simulink model "gm_sampleModel17924_sub"  (R2023b)
settings: Solver=VariableStepAuto  StartTime=0.0  StopTime=10.0  RelTol=1e-3
libraries: hdlsllib x3, simulink x2
settings Model: Creator=Tsmc  LastModifiedBy=Tsmc
settings OptimizationCC: BlockReduction=off  ConditionallyExecuteInputs=off
settings DebuggingCC: InheritedTsInSrcMsg=none

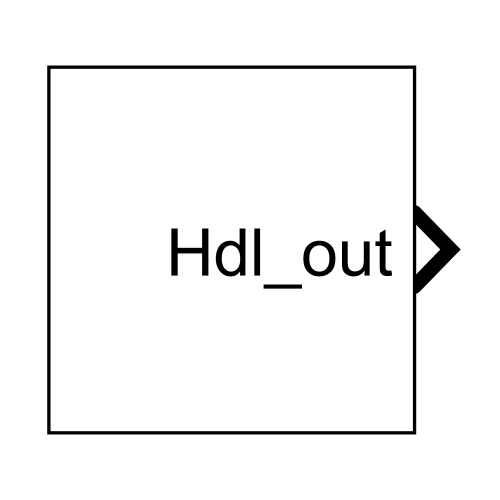
[thumbnail: Simulink's stored preview of the top-level diagram]
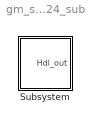
== system gm_sampleModel17924_sub ==
  Subsystem : Subsystem

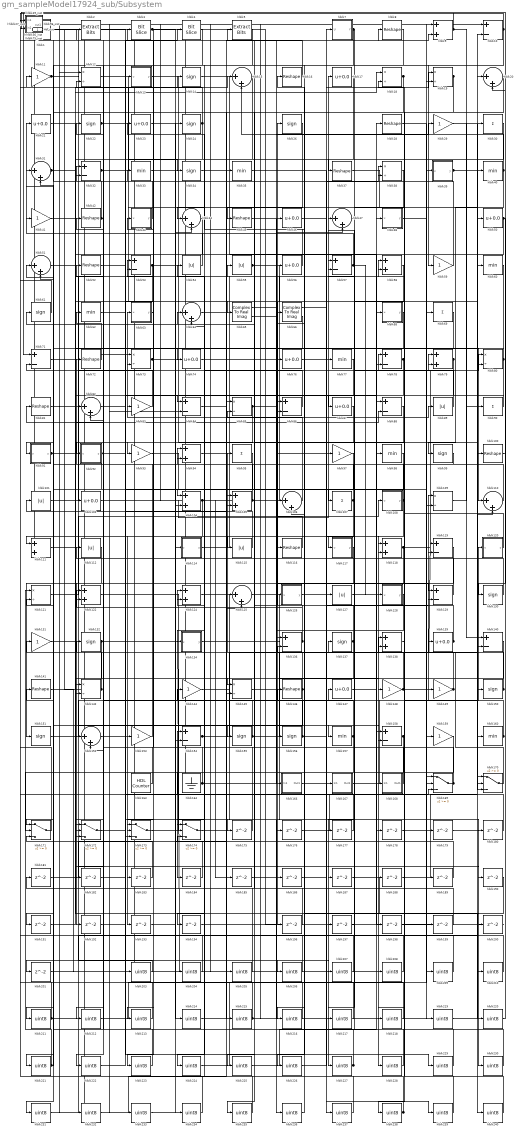
== system gm_sampleModel17924_sub/Subsystem ==
  hlblk1 : Subsystem  mask(Detect Rise Nonnegative){vinit=double(0), InputProcessing=Elements as channels (sample based), OutDataTypeStr=uint8}
      mask prompts: vinit "Simulink:masks:InitialCondition_MP"; InputProcessing "Simulink:masks:InputProcessing_MP"; OutDataTypeStr "Simulink:masks:OutputDataType_MP"
      mask help: Simulink:masks:DetectRiseNonnegative_MD
      mask init:
      | InputProcessing = 'Elements as channels (sample based)';
      | OutDataTypeStr = 'uint8';
      | vinit = double(0);
      mask TypeOptions InputProcessing: Simulink:masks:ColumnsAsChannelsFrameBased | Simulink:masks:ElementsAsChannelsSampleBased
      mask TypeOptions OutDataTypeStr: Simulink:masks:uint8 | Simulink:masks:boolean
      mask Display: fprintf('U >= 0\n&  NOT\nU/z >= 0')
  hlblk{10,32,53,57,71,78,84,86,88,119,129,136,140,154,158} (15 alike) : Sum  Inputs=+-  OutDataTypeStr=uint8
  hlblk{8,16,28,37,42,45,52,72,81,100,116,141,146} (13 alike) : Reshape
  hlblk{54..55,89,101,112,115,127} (7 alike) : Abs  OutDataTypeStr=uint8  SaturateOnIntegerOverflow=off
  hlblk{17,21,23,46,50,56,74,76,87,102,139,147} (12 alike) : Bias  Bias=0.0  SaturateOnIntegerOverflow=off
  hlblk{9,58,79,94,104..105,111,118,122,124,138} (11 alike) : Sum  OutDataTypeStr=uint8
  hlblk{15,20,31,44,47,51,64,82,106,110,125,152} (12 alike) : Sum  Inputs=|++  OutDataTypeStr=uint8
  hlblk{30,69,90,95,107} (5 alike) : Sum  Inputs=+  OutDataTypeStr=uint8
  hlblk108 : Subsystem  mask(Real World Value Increment){}
      mask help: Simulink:masks:RealWorldValueIncrement_MD
      mask Display: disp('V++')
  hlblk{12,18..19,38,73,80,85,109,121,142,145} (11 alike) : Product  Inputs=*/  OutDataTypeStr=uint8  RndMeth=Zero  SaturateOnIntegerOverflow=on
  hlblk{11,29,41,59,83,93,97,131,144,148..149,153,159} (13 alike) : Gain  OutDataTypeStr=uint8
  hlblk113_inst : Subsystem
  hlblk114 : Subsystem  mask(Real World Value Increment){}
      mask help: Simulink:masks:RealWorldValueIncrement_MD
      mask Display: disp('V++')
  hlblk117 : Subsystem  mask(Real World Value Increment){}
      mask help: Simulink:masks:RealWorldValueIncrement_MD
      mask Display: disp('V++')
  hlblk120 : Subsystem  mask(Real World Value Increment){}
      mask help: Simulink:masks:RealWorldValueIncrement_MD
      mask Display: disp('V++')
  hlblk126 : Subsystem  mask(Real World Value Increment){}
      mask help: Simulink:masks:RealWorldValueIncrement_MD
      mask Display: disp('V++')
  hlblk128 : Subsystem  mask(Real World Value Increment){}
      mask help: Simulink:masks:RealWorldValueIncrement_MD
      mask Display: disp('V++')
  hlblk13 : Subsystem  mask(Real World Value Increment){}
      mask help: Simulink:masks:RealWorldValueIncrement_MD
      mask Display: disp('V++')
  hlblk{14,22,24,26,34,61,99,130,132,137,150..151,155..156} (14 alike) : Signum
  hlblk133_inst : Subsystem
  hlblk134 : Subsystem  mask(Real World Value Increment){}
      mask help: Simulink:masks:RealWorldValueIncrement_MD
      mask Display: disp('V++')
  hlblk135_inst : Subsystem
  hlblk143_inst : Subsystem
  hlblk{33,35,40,60,62,77,98,157,160} (9 alike) : MinMax  OutDataTypeStr=uint8
  hlblk163 : hdlsllib/Sources/HDL Counter  CountType=Count limited  CountInit=0  CountStep=1  CountMax=25  CountFromType=Initial value  CountFrom=0  CountResetPort=off  CountLoadPort=off  CountEnbPort=off  CountDirPort=off  CountHitOutputPort=off  CountDataType=Unsigned  CountWordLen=8  CountFracLen=0  CountSampTime=1
  hlblk164 : Ground
  hlblk166 : Subsystem
  hlblk167 : Subsystem
  hlblk168 : Subsystem
  hlblk{169..174} (6 alike) : Switch  OutDataTypeStr=uint8  SaturateOnIntegerOverflow=off  InputSameDT=off
  hlblk{175..194,196..201} (26 alike) : Delay  SampleTime=1
  hlblk2 : simulink/Logic and Bit Operations/Extract Bits  bitsToExtract=Upper half  numBits=8  bitIdxRange=[0 7]  outScalingMode=Preserve fixed-point scaling
      settings: LibrarySourceBlock=|
      | hdlsllib/Logic and Bit
      | Operations/Extract Bits
  hlblk{203..240} (38 alike) : DataTypeConversion  OutDataTypeStr=uint8  SaturateOnIntegerOverflow=off  RndMeth=Floor
  hlblk25_inst : Subsystem
  hlblk27_inst : Subsystem
  hlblk3 : hdlsllib/Logic and Bit Operations/Bit Slice  lidx=7  ridx=0
  hlblk36_inst : Subsystem
  hlblk39 : Subsystem  mask(Real World Value Increment){}
      mask help: Simulink:masks:RealWorldValueIncrement_MD
      mask Display: disp('V++')
  hlblk4 : hdlsllib/Logic and Bit Operations/Bit Slice  lidx=7  ridx=0
  hlblk43 : Subsystem  mask(Real World Value Increment){}
      mask help: Simulink:masks:RealWorldValueIncrement_MD
      mask Display: disp('V++')
  hlblk48 : Subsystem  mask(Real World Value Increment){}
      mask help: Simulink:masks:RealWorldValueIncrement_MD
      mask Display: disp('V++')
  hlblk49_inst : Subsystem
  hlblk5 : simulink/Logic and Bit Operations/Extract Bits  bitsToExtract=Upper half  numBits=8  bitIdxRange=[0 7]  outScalingMode=Preserve fixed-point scaling
      settings: LibrarySourceBlock=|
      | hdlsllib/Logic and Bit
      | Operations/Extract Bits
  hlblk63 : Subsystem  mask(Real World Value Increment){}
      mask help: Simulink:masks:RealWorldValueIncrement_MD
      mask Display: disp('V++')
  hlblk65 : ComplexToRealImag
  hlblk66 : ComplexToRealImag
  hlblk68 : Subsystem  mask(Real World Value Increment){}
      mask help: Simulink:masks:RealWorldValueIncrement_MD
      mask Display: disp('V++')
  hlblk7 : Subsystem  mask(Detect Fall Negative){vinit=double(0), InputProcessing=Elements as channels (sample based), OutDataTypeStr=uint8}
      mask prompts: vinit "Simulink:masks:InitialCondition_MP"; InputProcessing "Simulink:masks:InputProcessing_MP"; OutDataTypeStr "Simulink:masks:OutputDataType_MP"
      mask help: Simulink:masks:DetectFallNegative_MD
      mask init:
      | InputProcessing = 'Elements as channels (sample based)';
      | OutDataTypeStr = 'uint8';
      | vinit = double(0);
      mask TypeOptions InputProcessing: Simulink:masks:ColumnsAsChannelsFrameBased | Simulink:masks:ElementsAsChannelsSampleBased
      mask TypeOptions OutDataTypeStr: Simulink:masks:uint8 | Simulink:masks:boolean
      mask Display: fprintf('U < 0\n&  NOT\nU/z < 0')
  hlblk75_inst : Subsystem
  hlblk91 : Subsystem  mask(Real World Value Increment){}
      mask help: Simulink:masks:RealWorldValueIncrement_MD
      mask Display: disp('V++')
  hlblk92 : Subsystem  mask(Real World Value Increment){}
      mask help: Simulink:masks:RealWorldValueIncrement_MD
      mask Display: disp('V++')
  hlblk96_inst : Subsystem
  Hdl_out : Outport  OutDataTypeStr=uint8  SampleTime=1
  wires:
  hlblk1/1(Y) -> hlblk206/1
  hlblk10/1 -> hlblk71/1, hlblk106/2, hlblk59/1
  hlblk100/1 -> hlblk75_inst/2(in2)
  hlblk101/1 -> hlblk55/1
  hlblk102/1 -> hlblk17/1
  hlblk104/1 -> hlblk111/1, hlblk185/1
  hlblk105/1 -> hlblk94/1, hlblk58/1
  hlblk106/1 -> hlblk63/1(u)
  hlblk107/1 -> hlblk31/2, hlblk193/1
  hlblk108/1(y) -> hlblk72/1, hlblk228/1
  hlblk109/1 -> hlblk30/1
  hlblk11/1 -> hlblk214/1, hlblk110/1
  hlblk110/1 -> hlblk5/1
  hlblk111/1 -> hlblk157/1
  hlblk112/1 -> hlblk151/1
  hlblk113_inst/1(out1) -> hlblk205/1
  hlblk114/1(y) -> hlblk48/1(u)
  hlblk115/1 -> hlblk51/1
  hlblk116/1 -> hlblk26/1
  hlblk117/1(y) -> hlblk183/1
  hlblk118/1 -> hlblk196/1, hlblk80/1
  hlblk119/1 -> hlblk192/1
  hlblk12/1 -> hlblk176/1
  hlblk120/1(y) -> hlblk18/2
  hlblk121/1 -> hlblk108/1(u)
  hlblk122/1 -> hlblk175/1
  hlblk124/1 -> hlblk227/1
  hlblk125/1 -> hlblk230/1
  hlblk126/1(y) -> hlblk7/1(U)
  hlblk127/1 -> hlblk68/1(u)
  hlblk128/1(y) -> hlblk136/1
  hlblk129/1 -> hlblk53/1
  hlblk13/1(y) -> hlblk170/2
  hlblk130/1 -> hlblk109/1
  hlblk131/1 -> hlblk187/1
  hlblk132/1 -> hlblk204/1, hlblk172/3
  hlblk133_inst/1(out1) -> hlblk111/2, hlblk167/1(In1)
  hlblk134/1(y) -> hlblk148/1
  hlblk135_inst/1(out1) -> hlblk12/1
  hlblk136/1 -> hlblk86/2, hlblk122/1
  hlblk137/1 -> hlblk235/1, hlblk83/1
  hlblk138/1 -> hlblk238/1
  hlblk139/1 -> hlblk61/1, hlblk112/1
  hlblk14/1 -> hlblk198/1
  hlblk140/1 -> hlblk142/2
  hlblk141/1 -> hlblk203/1
  hlblk142/1 -> hlblk131/1, Hdl_out/1
  hlblk143_inst/1(out1) -> hlblk84/2, hlblk234/1, hlblk220/1
  hlblk144/1 -> hlblk236/1
  hlblk145/1 -> hlblk28/1
  hlblk146/1 -> hlblk46/1, hlblk171/1, hlblk43/1(u)
  hlblk147/1 -> hlblk88/1
  hlblk148/1 -> hlblk119/1, hlblk95/1
  hlblk149/1 -> hlblk22/1, hlblk119/2
  hlblk15/1 -> hlblk194/1
  hlblk150/1 -> hlblk142/1, hlblk73/2
  hlblk151/1 -> hlblk120/1(u)
  hlblk152/1 -> hlblk153/1
  hlblk153/1 -> hlblk2/1
  hlblk154/1 -> hlblk147/1, hlblk140/2
  hlblk155/1 -> hlblk32/1, hlblk152/1, hlblk40/1
  hlblk156/1 -> hlblk3/1, hlblk129/2, hlblk38/1
  hlblk157/1 -> hlblk184/1, hlblk126/1(u)
  hlblk158/1 -> hlblk173/2, hlblk171/2
  hlblk159/1 -> hlblk223/1
  hlblk16/1 -> hlblk135_inst/2(in2)
  hlblk160/1 -> hlblk58/2, hlblk149/1
  hlblk163/1 -> hlblk52/1
  hlblk164/1 -> hlblk53/2, hlblk237/1
  hlblk166/1(Out1) -> hlblk19/1
  hlblk167/1(Out1) -> hlblk19/2
  hlblk168/1(Out1) -> hlblk47/1
  hlblk169/1 -> hlblk82/2, hlblk81/1, hlblk16/1
  hlblk17/1 -> hlblk37/1
  hlblk170/1 -> hlblk139/1
  hlblk171/1 -> hlblk143_inst/1(in1)
  hlblk172/1 -> hlblk105/1
  hlblk173/1 -> hlblk150/1
  hlblk174/1 -> hlblk89/1
  hlblk175/1 -> hlblk27_inst/2(in2)
  hlblk176/1 -> hlblk9/1
  hlblk177/1 -> hlblk154/1
  hlblk178/1 -> hlblk170/1
  hlblk179/1 -> hlblk210/1
  hlblk18/1 -> hlblk51/2, hlblk145/1
  hlblk180/1 -> hlblk25_inst/2(in2)
  hlblk181/1 -> hlblk105/2
  hlblk182/1 -> hlblk169/3
  hlblk183/1 -> hlblk121/2
  hlblk184/1 -> hlblk174/3
  hlblk185/1 -> hlblk86/1
  hlblk186/1 -> hlblk79/1
  hlblk187/1 -> hlblk240/1
  hlblk188/1 -> hlblk110/2
  hlblk189/1 -> hlblk174/2
  hlblk19/1 -> hlblk104/1, hlblk145/2
  hlblk190/1 -> hlblk216/1
  hlblk191/1 -> hlblk88/2
  hlblk192/1 -> hlblk80/2
  hlblk193/1 -> hlblk78/1
  hlblk194/1 -> hlblk47/2
  hlblk196/1 -> hlblk71/2
  hlblk197/1 -> hlblk57/1
  hlblk198/1 -> hlblk169/2
  hlblk199/1 -> hlblk85/2
  hlblk2/1 -> hlblk186/1
  hlblk20/1 -> hlblk218/1
  hlblk200/1 -> hlblk1/1(U)
  hlblk201/1 -> hlblk207/1
  hlblk203/1 -> hlblk201/1
  hlblk204/1 -> hlblk141/1
  hlblk205/1 -> hlblk85/1
  hlblk206/1 -> hlblk113_inst/1(in1)
  hlblk207/1 -> hlblk113_inst/2(in2)
  hlblk208/1 -> hlblk96_inst/1(in1)
  hlblk209/1 -> hlblk49_inst/1(in1)
  hlblk21/1 -> hlblk102/1
  hlblk210/1 -> hlblk49_inst/2(in2)
  hlblk211/1 -> hlblk24/1, hlblk133_inst/2(in2), hlblk10/2
  hlblk212/1 -> hlblk69/1
  hlblk213/1 -> hlblk143_inst/2(in2)
  hlblk214/1 -> hlblk98/1
  hlblk215/1 -> hlblk171/3, hlblk169/1
  hlblk216/1 -> hlblk64/1
  hlblk217/1 -> hlblk64/2
  hlblk218/1 -> hlblk135_inst/1(in1)
  hlblk219/1 -> hlblk20/1
  hlblk22/1 -> hlblk34/1, hlblk199/1
  hlblk220/1 -> hlblk20/2
  hlblk221/1 -> hlblk101/1, hlblk121/1
  hlblk222/1 -> hlblk4/1
  hlblk223/1 -> hlblk132/1
  hlblk224/1 -> hlblk159/1
  hlblk225/1 -> hlblk168/1(In1)
  hlblk226/1 -> hlblk77/1
  hlblk227/1 -> hlblk42/1, hlblk181/1
  hlblk228/1 -> hlblk124/1
  hlblk229/1 -> hlblk124/2
  hlblk23/1 -> hlblk44/2
  hlblk230/1 -> hlblk137/1
  hlblk231/1 -> hlblk125/1
  hlblk232/1 -> hlblk125/2
  hlblk233/1 -> hlblk114/1(u)
  hlblk234/1 -> hlblk36_inst/1(in1)
  hlblk235/1 -> hlblk36_inst/2(in2)
  hlblk236/1 -> hlblk146/1
  hlblk237/1 -> hlblk144/1
  hlblk238/1 -> hlblk66/1, hlblk136/2
  hlblk239/1 -> hlblk138/1
  hlblk24/1 -> hlblk96_inst/2(in2), hlblk32/2
  hlblk240/1 -> hlblk138/2
  hlblk25_inst/1(out1) -> hlblk232/1, hlblk10/1
  hlblk26/1 -> hlblk45/1
  hlblk27_inst/1(out1) -> hlblk13/1(u), hlblk35/1
  hlblk28/1 -> hlblk219/1
  hlblk29/1 -> hlblk60/1
  hlblk3/1 -> hlblk173/1, hlblk158/2
  hlblk30/1 -> hlblk172/1
  hlblk31/1 -> hlblk15/1, hlblk91/1(u)
  hlblk32/1 -> hlblk209/1, hlblk14/1
  hlblk33/1 -> hlblk190/1
  hlblk34/1 -> hlblk78/2
  hlblk35/1 -> hlblk239/1
  hlblk36_inst/1(out1) -> hlblk233/1
  hlblk37/1 -> hlblk160/1
  hlblk38/1 -> hlblk177/1
  hlblk39/1(y) -> hlblk50/1, hlblk90/1
  hlblk4/1 -> hlblk221/1
  hlblk40/1 -> hlblk99/1, hlblk15/2
  hlblk41/1 -> hlblk200/1
  hlblk42/1 -> hlblk152/2, hlblk133_inst/1(in1), hlblk12/2
  hlblk43/1(y) -> hlblk75_inst/1(in1)
  hlblk44/1 -> hlblk222/1
  hlblk45/1 -> hlblk156/1
  hlblk46/1 -> hlblk38/2
  hlblk47/1 -> hlblk217/1
  hlblk48/1(y) -> hlblk179/1
  hlblk49_inst/1(out1) -> hlblk208/1
  hlblk5/1 -> hlblk44/1
  hlblk50/1 -> hlblk172/2, hlblk130/1, hlblk118/2
  hlblk51/1 -> hlblk84/1
  hlblk52/1 -> hlblk65/1
  hlblk53/1 -> hlblk170/3, hlblk122/2
  hlblk54/1 -> hlblk21/1
  hlblk55/1 -> hlblk158/1, hlblk100/1, hlblk189/1
  hlblk56/1 -> hlblk23/1
  hlblk57/1 -> hlblk41/1, hlblk128/1(u)
  hlblk58/1 -> hlblk197/1
  hlblk59/1 -> hlblk11/1
  hlblk60/1 -> hlblk104/2
  hlblk61/1 -> hlblk25_inst/1(in1)
  hlblk62/1 -> hlblk180/1
  hlblk63/1(y) -> hlblk33/1
  hlblk64/1 -> hlblk215/1
  hlblk65/1 -> hlblk97/1
  hlblk65/2 -> hlblk29/1
  hlblk66/1 -> hlblk127/1
  hlblk66/2 -> hlblk224/1
  hlblk68/1(y) -> hlblk174/1
  hlblk69/1 -> hlblk211/1
  hlblk7/1(Y) -> hlblk182/1, hlblk117/1(u)
  hlblk71/1 -> hlblk76/1
  hlblk72/1 -> hlblk62/1
  hlblk73/1 -> hlblk188/1, hlblk166/1(In1)
  hlblk74/1 -> hlblk107/1
  hlblk75_inst/1(out1) -> hlblk106/1, hlblk73/1
  hlblk76/1 -> hlblk118/1
  hlblk77/1 -> hlblk225/1
  hlblk78/1 -> hlblk173/3, hlblk154/2
  hlblk79/1 -> hlblk116/1, hlblk115/1
  hlblk8/1 -> hlblk93/1
  hlblk80/1 -> hlblk74/1, hlblk134/1(u)
  hlblk81/1 -> hlblk39/1(u)
  hlblk82/1 -> hlblk109/2
  hlblk83/1 -> hlblk31/1
  hlblk84/1 -> hlblk8/1
  hlblk85/1 -> hlblk9/2, hlblk129/1, hlblk92/1(u)
  hlblk86/1 -> hlblk54/1
  hlblk87/1 -> hlblk155/1
  hlblk88/1 -> hlblk226/1
  hlblk89/1 -> hlblk57/2
  hlblk9/1 -> hlblk27_inst/1(in1), hlblk140/1
  hlblk90/1 -> hlblk87/1
  hlblk91/1(y) -> hlblk56/1, hlblk18/1
  hlblk92/1(y) -> hlblk231/1, hlblk229/1
  hlblk93/1 -> hlblk178/1
  hlblk94/1 -> hlblk79/2
  hlblk95/1 -> hlblk191/1
  hlblk96_inst/1(out1) -> hlblk82/1
  hlblk97/1 -> hlblk212/1
  hlblk98/1 -> hlblk213/1
  hlblk99/1 -> hlblk94/2

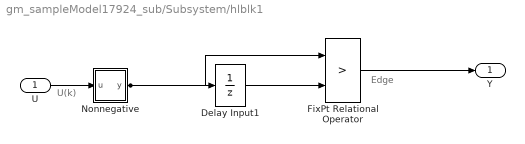
== system gm_sampleModel17924_sub/Subsystem/hlblk1 ==
  note: U(k)
  note: Edge
  U : Inport  OutDataTypeStr=uint8  SampleTime=1
  Delay Input1 : UnitDelay  Description=Store in Global RAM  DisableCoverage=on  InitialCondition=vinit  SampleTime=-1  HasFrameUpgradeWarning=on
  FixPt Relational Operator : RelationalOperator  Operator=>  OutDataTypeStr=fixdt(0, 8)  ZeroCross=off  InputSameDT=off
  Nonnegative : Subsystem  mask(Compare To Zero){relop=>=, OutDataTypeStr=boolean, ZeroCross=off}
      mask prompts: relop "Simulink:masks:Operator_MP"; OutDataTypeStr "Simulink:masks:OutputDataType_MP"; ZeroCross "Simulink:masks:EnableZerocrossingDetection_MP"
      mask help: Simulink:masks:CompareToZero_MD
      mask init:
      | OutDataTypeStr = 'boolean';
      | ZeroCross = 'off';
      | blkName = 'sampleModel17924_sub/Subsystem/hlblk1/Nonnegative';
      | relop = '>=';
      | setValue = 'boolean';
      mask TypeOptions relop: == | ~= | < | <= | >= | >
      mask TypeOptions OutDataTypeStr: Simulink:masks:uint8 | Simulink:masks:boolean
      mask Callback ZeroCross: sl('zeroCrossEnable', gcbh);
      mask Display: disp([relop,' 0'])
  Y : Outport  SampleTime=1
  wires:
  U/1 -> Nonnegative/1(u)
  Delay Input1/1 -> FixPt Relational Operator/2
  FixPt Relational Operator/1 -> Y/1
  Nonnegative/1(y) -> FixPt Relational Operator/1, Delay Input1/1

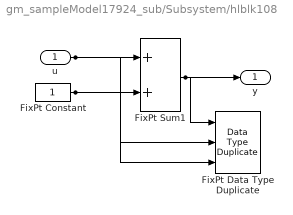
== system gm_sampleModel17924_sub/Subsystem/hlblk108 ==
  u : Inport  OutDataTypeStr=uint8  SampleTime=1
  FixPt Constant : Constant  DisableCoverage=on  OutDataTypeStr=Inherit: Inherit via back propagation  SampleTime=-1
  FixPt Data Type Duplicate : DataTypeDuplicate  DisableCoverage=on  NumInputPorts=3
  FixPt Sum1 : Sum  OutDataTypeStr=Inherit: Inherit via back propagation  InputSameDT=on  LockScale=on
  y : Outport  SampleTime=1
  wires:
  u/1 -> FixPt Sum1/1, FixPt Data Type Duplicate/2
  FixPt Constant/1 -> FixPt Sum1/2, FixPt Data Type Duplicate/3
  FixPt Sum1/1 -> FixPt Data Type Duplicate/1, y/1

== system gm_sampleModel17924_sub/Subsystem/hlblk113_inst ==
  in1 : Inport  OutDataTypeStr=uint8  SampleTime=1
  in2 : Inport  Port=2  OutDataTypeStr=uint8  SampleTime=1
  mul_hlblk113_dotp_mulcomp : Product  Inputs=**  OutDataTypeStr=uint8  SampleTime=1
  out1 : Outport  OutDataTypeStr=uint8  SampleTime=1
  wires:
  in1/1 -> mul_hlblk113_dotp_mulcomp/1
  in2/1 -> mul_hlblk113_dotp_mulcomp/2
  mul_hlblk113_dotp_mulcomp/1 -> out1/1

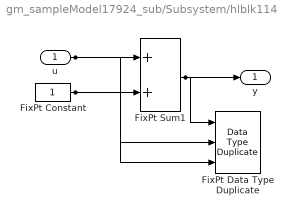
== system gm_sampleModel17924_sub/Subsystem/hlblk114 ==
  u : Inport  OutDataTypeStr=uint8  SampleTime=1
  FixPt Constant : Constant  DisableCoverage=on  OutDataTypeStr=Inherit: Inherit via back propagation  SampleTime=-1
  FixPt Data Type Duplicate : DataTypeDuplicate  DisableCoverage=on  NumInputPorts=3
  FixPt Sum1 : Sum  OutDataTypeStr=Inherit: Inherit via back propagation  InputSameDT=on  LockScale=on
  y : Outport  SampleTime=1
  wires:
  u/1 -> FixPt Sum1/1, FixPt Data Type Duplicate/2
  FixPt Constant/1 -> FixPt Sum1/2, FixPt Data Type Duplicate/3
  FixPt Sum1/1 -> FixPt Data Type Duplicate/1, y/1

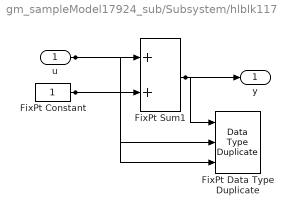
== system gm_sampleModel17924_sub/Subsystem/hlblk117 ==
  u : Inport  OutDataTypeStr=uint8  SampleTime=1
  FixPt Constant : Constant  DisableCoverage=on  OutDataTypeStr=Inherit: Inherit via back propagation  SampleTime=-1
  FixPt Data Type Duplicate : DataTypeDuplicate  DisableCoverage=on  NumInputPorts=3
  FixPt Sum1 : Sum  OutDataTypeStr=Inherit: Inherit via back propagation  InputSameDT=on  LockScale=on
  y : Outport  SampleTime=1
  wires:
  u/1 -> FixPt Sum1/1, FixPt Data Type Duplicate/2
  FixPt Constant/1 -> FixPt Sum1/2, FixPt Data Type Duplicate/3
  FixPt Sum1/1 -> FixPt Data Type Duplicate/1, y/1

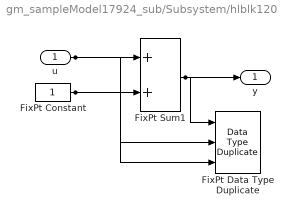
== system gm_sampleModel17924_sub/Subsystem/hlblk120 ==
  u : Inport  OutDataTypeStr=uint8  SampleTime=1
  FixPt Constant : Constant  DisableCoverage=on  OutDataTypeStr=Inherit: Inherit via back propagation  SampleTime=-1
  FixPt Data Type Duplicate : DataTypeDuplicate  DisableCoverage=on  NumInputPorts=3
  FixPt Sum1 : Sum  OutDataTypeStr=Inherit: Inherit via back propagation  InputSameDT=on  LockScale=on
  y : Outport  SampleTime=1
  wires:
  u/1 -> FixPt Sum1/1, FixPt Data Type Duplicate/2
  FixPt Constant/1 -> FixPt Sum1/2, FixPt Data Type Duplicate/3
  FixPt Sum1/1 -> FixPt Data Type Duplicate/1, y/1

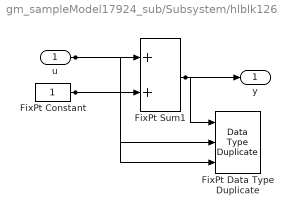
== system gm_sampleModel17924_sub/Subsystem/hlblk126 ==
  u : Inport  OutDataTypeStr=uint8  SampleTime=1
  FixPt Constant : Constant  DisableCoverage=on  OutDataTypeStr=Inherit: Inherit via back propagation  SampleTime=-1
  FixPt Data Type Duplicate : DataTypeDuplicate  DisableCoverage=on  NumInputPorts=3
  FixPt Sum1 : Sum  OutDataTypeStr=Inherit: Inherit via back propagation  InputSameDT=on  LockScale=on
  y : Outport  SampleTime=1
  wires:
  u/1 -> FixPt Sum1/1, FixPt Data Type Duplicate/2
  FixPt Constant/1 -> FixPt Sum1/2, FixPt Data Type Duplicate/3
  FixPt Sum1/1 -> FixPt Data Type Duplicate/1, y/1

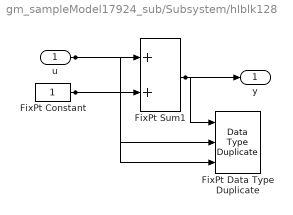
== system gm_sampleModel17924_sub/Subsystem/hlblk128 ==
  u : Inport  OutDataTypeStr=uint8  SampleTime=1
  FixPt Constant : Constant  DisableCoverage=on  OutDataTypeStr=Inherit: Inherit via back propagation  SampleTime=-1
  FixPt Data Type Duplicate : DataTypeDuplicate  DisableCoverage=on  NumInputPorts=3
  FixPt Sum1 : Sum  OutDataTypeStr=Inherit: Inherit via back propagation  InputSameDT=on  LockScale=on
  y : Outport  SampleTime=1
  wires:
  u/1 -> FixPt Sum1/1, FixPt Data Type Duplicate/2
  FixPt Constant/1 -> FixPt Sum1/2, FixPt Data Type Duplicate/3
  FixPt Sum1/1 -> FixPt Data Type Duplicate/1, y/1

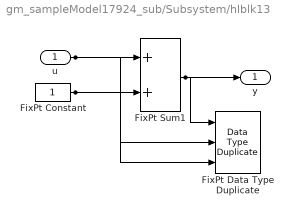
== system gm_sampleModel17924_sub/Subsystem/hlblk13 ==
  u : Inport  OutDataTypeStr=uint8  SampleTime=1
  FixPt Constant : Constant  DisableCoverage=on  OutDataTypeStr=Inherit: Inherit via back propagation  SampleTime=-1
  FixPt Data Type Duplicate : DataTypeDuplicate  DisableCoverage=on  NumInputPorts=3
  FixPt Sum1 : Sum  OutDataTypeStr=Inherit: Inherit via back propagation  InputSameDT=on  LockScale=on
  y : Outport  SampleTime=1
  wires:
  u/1 -> FixPt Sum1/1, FixPt Data Type Duplicate/2
  FixPt Constant/1 -> FixPt Sum1/2, FixPt Data Type Duplicate/3
  FixPt Sum1/1 -> FixPt Data Type Duplicate/1, y/1

== system gm_sampleModel17924_sub/Subsystem/hlblk133_inst ==
  in1 : Inport  OutDataTypeStr=uint8  SampleTime=1
  in2 : Inport  Port=2  OutDataTypeStr=uint8  SampleTime=1
  mul_hlblk133_dotp_mulcomp : Product  Inputs=**  OutDataTypeStr=uint8  SampleTime=1
  out1 : Outport  OutDataTypeStr=uint8  SampleTime=1
  wires:
  in1/1 -> mul_hlblk133_dotp_mulcomp/1
  in2/1 -> mul_hlblk133_dotp_mulcomp/2
  mul_hlblk133_dotp_mulcomp/1 -> out1/1

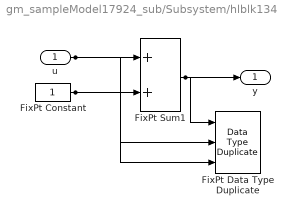
== system gm_sampleModel17924_sub/Subsystem/hlblk134 ==
  u : Inport  OutDataTypeStr=uint8  SampleTime=1
  FixPt Constant : Constant  DisableCoverage=on  OutDataTypeStr=Inherit: Inherit via back propagation  SampleTime=-1
  FixPt Data Type Duplicate : DataTypeDuplicate  DisableCoverage=on  NumInputPorts=3
  FixPt Sum1 : Sum  OutDataTypeStr=Inherit: Inherit via back propagation  InputSameDT=on  LockScale=on
  y : Outport  SampleTime=1
  wires:
  u/1 -> FixPt Sum1/1, FixPt Data Type Duplicate/2
  FixPt Constant/1 -> FixPt Sum1/2, FixPt Data Type Duplicate/3
  FixPt Sum1/1 -> FixPt Data Type Duplicate/1, y/1

== system gm_sampleModel17924_sub/Subsystem/hlblk135_inst ==
  in1 : Inport  OutDataTypeStr=uint8  SampleTime=1
  in2 : Inport  Port=2  OutDataTypeStr=uint8  SampleTime=1
  mul_hlblk135_dotp_mulcomp : Product  Inputs=**  OutDataTypeStr=uint8  SampleTime=1
  out1 : Outport  OutDataTypeStr=uint8  SampleTime=1
  wires:
  in1/1 -> mul_hlblk135_dotp_mulcomp/1
  in2/1 -> mul_hlblk135_dotp_mulcomp/2
  mul_hlblk135_dotp_mulcomp/1 -> out1/1

== system gm_sampleModel17924_sub/Subsystem/hlblk143_inst ==
  in1 : Inport  OutDataTypeStr=uint8  SampleTime=1
  in2 : Inport  Port=2  OutDataTypeStr=uint8  SampleTime=1
  mul_hlblk143_dotp_mulcomp : Product  Inputs=**  OutDataTypeStr=uint8  SampleTime=1
  out1 : Outport  OutDataTypeStr=uint8  SampleTime=1
  wires:
  in1/1 -> mul_hlblk143_dotp_mulcomp/1
  in2/1 -> mul_hlblk143_dotp_mulcomp/2
  mul_hlblk143_dotp_mulcomp/1 -> out1/1

== system gm_sampleModel17924_sub/Subsystem/hlblk166 ==
  In1 : Inport  OutDataTypeStr=uint8  PortDimensions=1  SampleTime=1
  Out1 : Outport  SampleTime=1
  wires:
  In1/1 -> Out1/1

== system gm_sampleModel17924_sub/Subsystem/hlblk167 ==
  In1 : Inport  OutDataTypeStr=uint8  PortDimensions=1  SampleTime=1
  Out1 : Outport  SampleTime=1
  wires:
  In1/1 -> Out1/1

== system gm_sampleModel17924_sub/Subsystem/hlblk168 ==
  In1 : Inport  OutDataTypeStr=uint8  PortDimensions=1  SampleTime=1
  Out1 : Outport  SampleTime=1
  wires:
  In1/1 -> Out1/1

== system gm_sampleModel17924_sub/Subsystem/hlblk25_inst ==
  in1 : Inport  OutDataTypeStr=uint8  SampleTime=1
  in2 : Inport  Port=2  OutDataTypeStr=uint8  SampleTime=1
  mul_hlblk25_dotp_mulcomp : Product  Inputs=**  OutDataTypeStr=uint8  SampleTime=1
  out1 : Outport  OutDataTypeStr=uint8  SampleTime=1
  wires:
  in1/1 -> mul_hlblk25_dotp_mulcomp/1
  in2/1 -> mul_hlblk25_dotp_mulcomp/2
  mul_hlblk25_dotp_mulcomp/1 -> out1/1

== system gm_sampleModel17924_sub/Subsystem/hlblk27_inst ==
  in1 : Inport  OutDataTypeStr=uint8  SampleTime=1
  in2 : Inport  Port=2  OutDataTypeStr=uint8  SampleTime=1
  mul_hlblk27_dotp_mulcomp : Product  Inputs=**  OutDataTypeStr=uint8  SampleTime=1
  out1 : Outport  OutDataTypeStr=uint8  SampleTime=1
  wires:
  in1/1 -> mul_hlblk27_dotp_mulcomp/1
  in2/1 -> mul_hlblk27_dotp_mulcomp/2
  mul_hlblk27_dotp_mulcomp/1 -> out1/1

== system gm_sampleModel17924_sub/Subsystem/hlblk36_inst ==
  in1 : Inport  OutDataTypeStr=uint8  SampleTime=1
  in2 : Inport  Port=2  OutDataTypeStr=uint8  SampleTime=1
  mul_hlblk36_dotp_mulcomp : Product  Inputs=**  OutDataTypeStr=uint8  SampleTime=1
  out1 : Outport  OutDataTypeStr=uint8  SampleTime=1
  wires:
  in1/1 -> mul_hlblk36_dotp_mulcomp/1
  in2/1 -> mul_hlblk36_dotp_mulcomp/2
  mul_hlblk36_dotp_mulcomp/1 -> out1/1

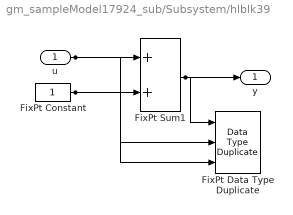
== system gm_sampleModel17924_sub/Subsystem/hlblk39 ==
  u : Inport  OutDataTypeStr=uint8  SampleTime=1
  FixPt Constant : Constant  DisableCoverage=on  OutDataTypeStr=Inherit: Inherit via back propagation  SampleTime=-1
  FixPt Data Type Duplicate : DataTypeDuplicate  DisableCoverage=on  NumInputPorts=3
  FixPt Sum1 : Sum  OutDataTypeStr=Inherit: Inherit via back propagation  InputSameDT=on  LockScale=on
  y : Outport  SampleTime=1
  wires:
  u/1 -> FixPt Sum1/1, FixPt Data Type Duplicate/2
  FixPt Constant/1 -> FixPt Sum1/2, FixPt Data Type Duplicate/3
  FixPt Sum1/1 -> FixPt Data Type Duplicate/1, y/1

== system gm_sampleModel17924_sub/Subsystem/hlblk43 ==
  u : Inport  OutDataTypeStr=uint8  SampleTime=1
  FixPt Constant : Constant  DisableCoverage=on  OutDataTypeStr=Inherit: Inherit via back propagation  SampleTime=-1
  FixPt Data Type Duplicate : DataTypeDuplicate  DisableCoverage=on  NumInputPorts=3
  FixPt Sum1 : Sum  OutDataTypeStr=Inherit: Inherit via back propagation  InputSameDT=on  LockScale=on
  y : Outport  SampleTime=1
  wires:
  u/1 -> FixPt Sum1/1, FixPt Data Type Duplicate/2
  FixPt Constant/1 -> FixPt Sum1/2, FixPt Data Type Duplicate/3
  FixPt Sum1/1 -> FixPt Data Type Duplicate/1, y/1

== system gm_sampleModel17924_sub/Subsystem/hlblk48 ==
  u : Inport  OutDataTypeStr=uint8  SampleTime=1
  FixPt Constant : Constant  DisableCoverage=on  OutDataTypeStr=Inherit: Inherit via back propagation  SampleTime=-1
  FixPt Data Type Duplicate : DataTypeDuplicate  DisableCoverage=on  NumInputPorts=3
  FixPt Sum1 : Sum  OutDataTypeStr=Inherit: Inherit via back propagation  InputSameDT=on  LockScale=on
  y : Outport  SampleTime=1
  wires:
  u/1 -> FixPt Sum1/1, FixPt Data Type Duplicate/2
  FixPt Constant/1 -> FixPt Sum1/2, FixPt Data Type Duplicate/3
  FixPt Sum1/1 -> FixPt Data Type Duplicate/1, y/1

== system gm_sampleModel17924_sub/Subsystem/hlblk49_inst ==
  in1 : Inport  OutDataTypeStr=uint8  SampleTime=1
  in2 : Inport  Port=2  OutDataTypeStr=uint8  SampleTime=1
  mul_hlblk49_dotp_mulcomp : Product  Inputs=**  OutDataTypeStr=uint8  SampleTime=1
  out1 : Outport  OutDataTypeStr=uint8  SampleTime=1
  wires:
  in1/1 -> mul_hlblk49_dotp_mulcomp/1
  in2/1 -> mul_hlblk49_dotp_mulcomp/2
  mul_hlblk49_dotp_mulcomp/1 -> out1/1

== system gm_sampleModel17924_sub/Subsystem/hlblk63 ==
  u : Inport  OutDataTypeStr=uint8  SampleTime=1
  FixPt Constant : Constant  DisableCoverage=on  OutDataTypeStr=Inherit: Inherit via back propagation  SampleTime=-1
  FixPt Data Type Duplicate : DataTypeDuplicate  DisableCoverage=on  NumInputPorts=3
  FixPt Sum1 : Sum  OutDataTypeStr=Inherit: Inherit via back propagation  InputSameDT=on  LockScale=on
  y : Outport  SampleTime=1
  wires:
  u/1 -> FixPt Sum1/1, FixPt Data Type Duplicate/2
  FixPt Constant/1 -> FixPt Sum1/2, FixPt Data Type Duplicate/3
  FixPt Sum1/1 -> FixPt Data Type Duplicate/1, y/1

== system gm_sampleModel17924_sub/Subsystem/hlblk68 ==
  u : Inport  OutDataTypeStr=uint8  SampleTime=1
  FixPt Constant : Constant  DisableCoverage=on  OutDataTypeStr=Inherit: Inherit via back propagation  SampleTime=-1
  FixPt Data Type Duplicate : DataTypeDuplicate  DisableCoverage=on  NumInputPorts=3
  FixPt Sum1 : Sum  OutDataTypeStr=Inherit: Inherit via back propagation  InputSameDT=on  LockScale=on
  y : Outport  SampleTime=1
  wires:
  u/1 -> FixPt Sum1/1, FixPt Data Type Duplicate/2
  FixPt Constant/1 -> FixPt Sum1/2, FixPt Data Type Duplicate/3
  FixPt Sum1/1 -> FixPt Data Type Duplicate/1, y/1

== system gm_sampleModel17924_sub/Subsystem/hlblk7 ==
  note: U(k)
  note: Edge
  U : Inport  OutDataTypeStr=uint8  SampleTime=1
  Delay Input1 : UnitDelay  Description=Store in Global RAM  DisableCoverage=on  InitialCondition=vinit  SampleTime=-1  HasFrameUpgradeWarning=on
  FixPt Relational Operator : RelationalOperator  Operator=>  OutDataTypeStr=fixdt(0, 8)  ZeroCross=off  InputSameDT=off
  Negative : Subsystem  mask(Compare To Zero){relop=<, OutDataTypeStr=boolean, ZeroCross=off}
      mask prompts: relop "Simulink:masks:Operator_MP"; OutDataTypeStr "Simulink:masks:OutputDataType_MP"; ZeroCross "Simulink:masks:EnableZerocrossingDetection_MP"
      mask help: Simulink:masks:CompareToZero_MD
      mask init:
      | OutDataTypeStr = 'boolean';
      | ZeroCross = 'off';
      | blkName = 'sampleModel17924_sub/Subsystem/hlblk7/Negative';
      | relop = '<';
      | setValue = 'boolean';
      mask TypeOptions relop: == | ~= | < | <= | >= | >
      mask TypeOptions OutDataTypeStr: Simulink:masks:uint8 | Simulink:masks:boolean
      mask Callback ZeroCross: sl('zeroCrossEnable', gcbh);
      mask Display: disp([relop,' 0'])
  Y : Outport  SampleTime=1
  wires:
  U/1 -> Negative/1(u)
  Delay Input1/1 -> FixPt Relational Operator/2
  FixPt Relational Operator/1 -> Y/1
  Negative/1(y) -> FixPt Relational Operator/1, Delay Input1/1

== system gm_sampleModel17924_sub/Subsystem/hlblk75_inst ==
  in1 : Inport  OutDataTypeStr=uint8  SampleTime=1
  in2 : Inport  Port=2  OutDataTypeStr=uint8  SampleTime=1
  mul_hlblk75_dotp_mulcomp : Product  Inputs=**  OutDataTypeStr=uint8  SampleTime=1
  out1 : Outport  OutDataTypeStr=uint8  SampleTime=1
  wires:
  in1/1 -> mul_hlblk75_dotp_mulcomp/1
  in2/1 -> mul_hlblk75_dotp_mulcomp/2
  mul_hlblk75_dotp_mulcomp/1 -> out1/1

== system gm_sampleModel17924_sub/Subsystem/hlblk91 ==
  u : Inport  OutDataTypeStr=uint8  SampleTime=1
  FixPt Constant : Constant  DisableCoverage=on  OutDataTypeStr=Inherit: Inherit via back propagation  SampleTime=-1
  FixPt Data Type Duplicate : DataTypeDuplicate  DisableCoverage=on  NumInputPorts=3
  FixPt Sum1 : Sum  OutDataTypeStr=Inherit: Inherit via back propagation  InputSameDT=on  LockScale=on
  y : Outport  SampleTime=1
  wires:
  u/1 -> FixPt Sum1/1, FixPt Data Type Duplicate/2
  FixPt Constant/1 -> FixPt Sum1/2, FixPt Data Type Duplicate/3
  FixPt Sum1/1 -> FixPt Data Type Duplicate/1, y/1

== system gm_sampleModel17924_sub/Subsystem/hlblk92 ==
  u : Inport  OutDataTypeStr=uint8  SampleTime=1
  FixPt Constant : Constant  DisableCoverage=on  OutDataTypeStr=Inherit: Inherit via back propagation  SampleTime=-1
  FixPt Data Type Duplicate : DataTypeDuplicate  DisableCoverage=on  NumInputPorts=3
  FixPt Sum1 : Sum  OutDataTypeStr=Inherit: Inherit via back propagation  InputSameDT=on  LockScale=on
  y : Outport  SampleTime=1
  wires:
  u/1 -> FixPt Sum1/1, FixPt Data Type Duplicate/2
  FixPt Constant/1 -> FixPt Sum1/2, FixPt Data Type Duplicate/3
  FixPt Sum1/1 -> FixPt Data Type Duplicate/1, y/1

== system gm_sampleModel17924_sub/Subsystem/hlblk96_inst ==
  in1 : Inport  OutDataTypeStr=uint8  SampleTime=1
  in2 : Inport  Port=2  OutDataTypeStr=uint8  SampleTime=1
  mul_hlblk96_dotp_mulcomp : Product  Inputs=**  OutDataTypeStr=uint8  SampleTime=1
  out1 : Outport  OutDataTypeStr=uint8  SampleTime=1
  wires:
  in1/1 -> mul_hlblk96_dotp_mulcomp/1
  in2/1 -> mul_hlblk96_dotp_mulcomp/2
  mul_hlblk96_dotp_mulcomp/1 -> out1/1

== system gm_sampleModel17924_sub/Subsystem/hlblk1/Nonnegative ==
  u : Inport  OutDataTypeStr=uint8  SampleTime=1
  Compare : RelationalOperator  OutDataTypeStr=boolean  ZeroCross=off
  Constant : Constant  DisableCoverage=on  Value=0  OutDataTypeStr=Inherit: Inherit via back propagation  SampleTime=-1  PreserveConstantTs=on
  y : Outport  SampleTime=1
  wires:
  u/1 -> Compare/1
  Compare/1 -> y/1
  Constant/1 -> Compare/2

== system gm_sampleModel17924_sub/Subsystem/hlblk7/Negative ==
  u : Inport  OutDataTypeStr=uint8  SampleTime=1
  Compare : RelationalOperator  Operator=<  OutDataTypeStr=boolean  ZeroCross=off
  Constant : Constant  DisableCoverage=on  Value=0  OutDataTypeStr=Inherit: Inherit via back propagation  SampleTime=-1  PreserveConstantTs=on
  y : Outport  SampleTime=1
  wires:
  u/1 -> Compare/1
  Compare/1 -> y/1
  Constant/1 -> Compare/2
